simulink model "Mann_heat_transform"  (R2023a)
settings: Solver=VariableStepAuto  StartTime=0.0  StopTime=10.0  RelTol=1e-3
settings Model: Creator=bulldize  LastModifiedBy=bulldize

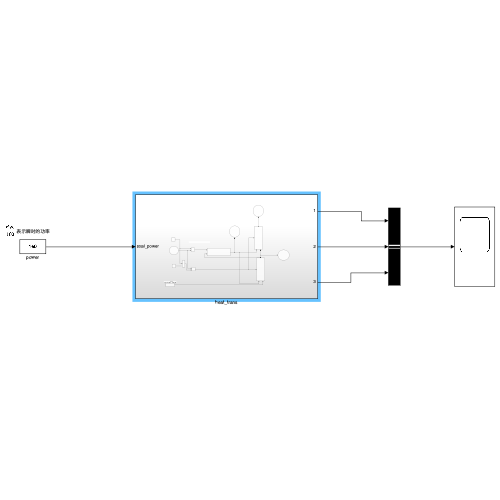
[thumbnail: Simulink's stored preview of the top-level diagram]
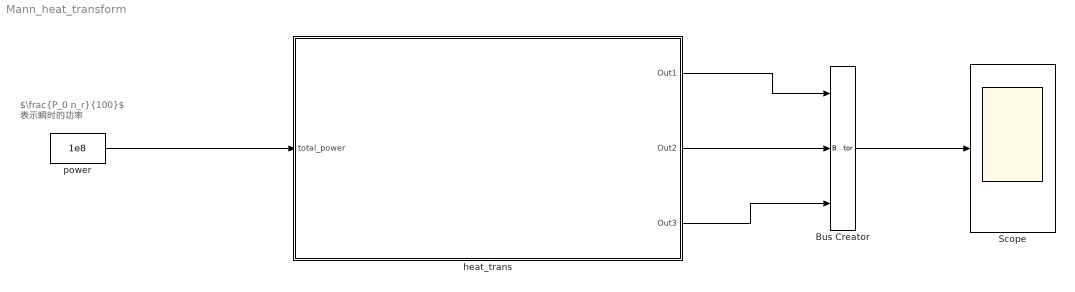
== system Mann_heat_transform ==
  note: $\frac{P_0 n_r}{100}$ 表示瞬时的功率
  Bus Creator : BusCreator  Inputs=3
  Scope : Scope
  heat_trans : Subsystem
  power : Constant  Value=1e8
  wires:
  power/1 -> heat_trans/1(total_power)
  heat_trans/1(Out1) -> Bus Creator/1
  heat_trans/2(Out2) -> Bus Creator/2
  heat_trans/3(Out3) -> Bus Creator/3
  Bus Creator/1 -> Scope/1

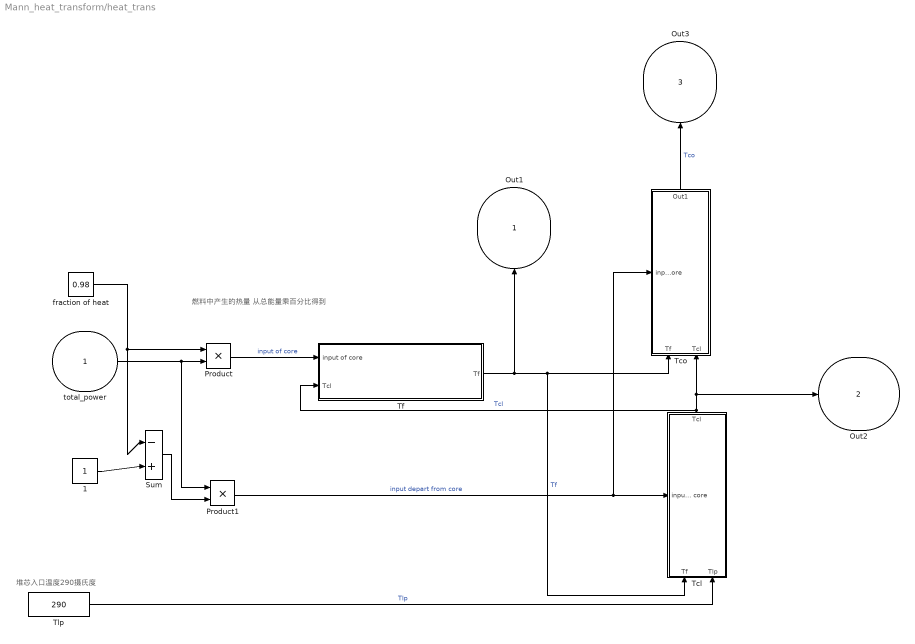
== system Mann_heat_transform/heat_trans ==
  note: 堆芯入口温度290摄氏度
  note: 燃料中产生的热量 从总能量乘百分比得到
  total_power : Inport
  1 : Constant
  Product : Product
  Product1 : Product
  Sum : Sum  Inputs=|-+
  Tcl : Subsystem
      settings: PortSchema="{\"entries\":[{\"content\":{\"sides\":[{\"content\":{\"connectorIds\":[\"In1\",\"In2\"]},\"type\":\"ConnectorPlacement.EquallySpacedRectSide\",\"uuid\":\"cb92287a-58d5-46bc-8bcc-fd7670e170d2\"},{\"content\":{\"connectorIds\":[\"Out1\"],\"side\":\"RIGHT\"},\"type\":\"ConnectorPlacement.EquallySpacedRectSide\",\"uuid\":\"3ab69de5-3a88-429e-9ba8-55afb0ea25a3\"},{\"content\":{\"connectorIds\":[\"In3\"],\"side\":\"TOP\"},\"type\":\"ConnectorPlacement.EquallySpacedRectSide\",\"uuid\":\"730caed0-fe0b-4665-bcfb-96be08a17aee\"}]},\"type\":\"ConnectorPlacement.EquallySpacedConnector\",\"uuid\":\"27471c3a-4cb2-4103-a1ca-5887cde1e89e\"}],\"packageUris\":[\"http://schema.mathworks.com/mf0/Connector/R2020b\"],\"version\":\"1.0\"}"
  Tco : Subsystem
      settings: PortSchema="{\"entries\":[{\"content\":{\"sides\":[{\"content\":{\"connectorIds\":[\"In1\",\"In2\"]},\"type\":\"ConnectorPlacement.EquallySpacedRectSide\",\"uuid\":\"cb92287a-58d5-46bc-8bcc-fd7670e170d2\"},{\"content\":{\"connectorIds\":[\"Out1\"],\"side\":\"RIGHT\"},\"type\":\"ConnectorPlacement.EquallySpacedRectSide\",\"uuid\":\"3ab69de5-3a88-429e-9ba8-55afb0ea25a3\"},{\"content\":{\"connectorIds\":[\"In3\"],\"side\":\"TOP\"},\"type\":\"ConnectorPlacement.EquallySpacedRectSide\",\"uuid\":\"730caed0-fe0b-4665-bcfb-96be08a17aee\"}]},\"type\":\"ConnectorPlacement.EquallySpacedConnector\",\"uuid\":\"27471c3a-4cb2-4103-a1ca-5887cde1e89e\"}],\"packageUris\":[\"http://schema.mathworks.com/mf0/Connector/R2020b\"],\"version\":\"1.0\"}"
  Tf : Subsystem
  Tlp : Constant  Value=290
  fraction of heat : Constant  Value=0.98
  Out1 : Outport
  Out2 : Outport  Port=2
  Out3 : Outport  Port=3
  wires:
  fraction of heat/1 -> Sum/1, Product/1
  total_power/1 -> Product1/1, Product/2
  1/1 -> Sum/2
  Sum/1 -> Product1/2
  Product/1 -> Tf/1(input of core)  "input of core"
  Tcl/1(Tcl) -> Tf/2(Tcl), Tco/2(Tcl), Out2/1  "Tcl"
  Tf/1(Tf) -> Tco/1(Tf), Tcl/1(Tf), Out1/1  "Tf"
  Tlp/1 -> Tcl/2(Tlp)  "Tlp"
  Product1/1 -> Tco/3(input depart from core), Tcl/3(input depart from core)  "input depart from core"
  Tco/1(Out1) -> Out3/1  "Tco"

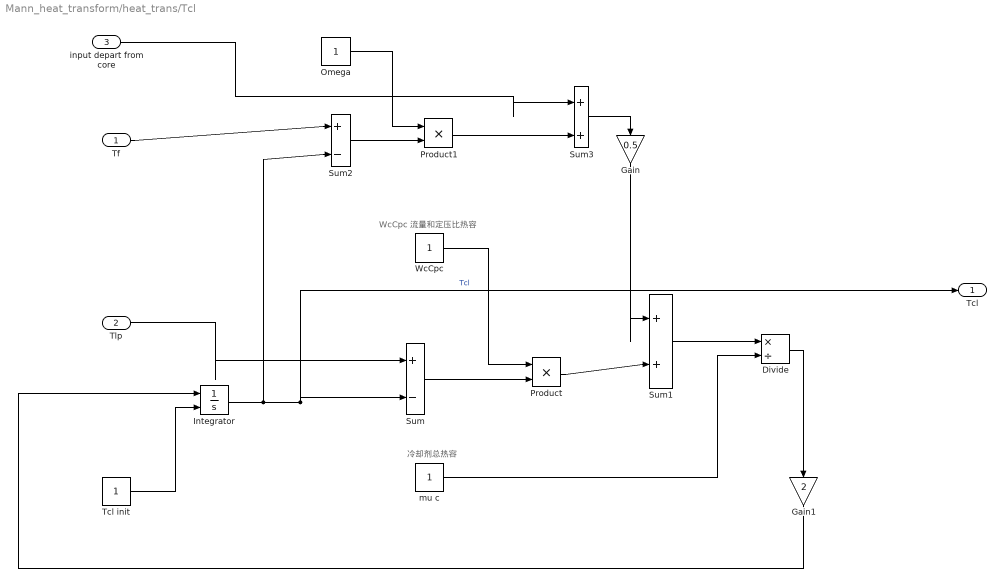
== system Mann_heat_transform/heat_trans/Tcl ==
  note: 冷却剂总热容
  note: WcCpc 流量和定压比热容
  Tf : Inport
  Tlp : Inport  Port=2
  input depart from core : Inport  Port=3
  Divide : Product  Inputs=*/
  Gain : Gain  Gain=0.5
  Gain1 : Gain  Gain=2
  Integrator : Integrator  InitialConditionSource=external
  Omega : Constant
  Product : Product
  Product1 : Product
  Sum : Sum  Inputs=|+-
  Sum1 : Sum  Inputs=|++
  Sum2 : Sum  Inputs=|+-
  Sum3 : Sum  Inputs=|++
  "Tcl init " : Constant
  WcCpc : Constant
  mu c : Constant
  Tcl : Outport
  wires:
  WcCpc/1 -> Product/1
  Product/1 -> Sum1/2
  "Tcl init "/1 -> Integrator/2
  Sum/1 -> Product/2
  Tlp/1 -> Sum/1
  Divide/1 -> Gain1/1
  Tf/1 -> Sum2/1
  Sum3/1 -> Gain/1
  mu c/1 -> Divide/2
  Integrator/1 -> Sum2/2, Tcl/1, Sum/2  "Tcl"
  Gain/1 -> Sum1/1
  Gain1/1 -> Integrator/1
  Sum1/1 -> Divide/1
  Omega/1 -> Product1/1
  Product1/1 -> Sum3/2
  Sum2/1 -> Product1/2
  input depart from core/1 -> Sum3/1

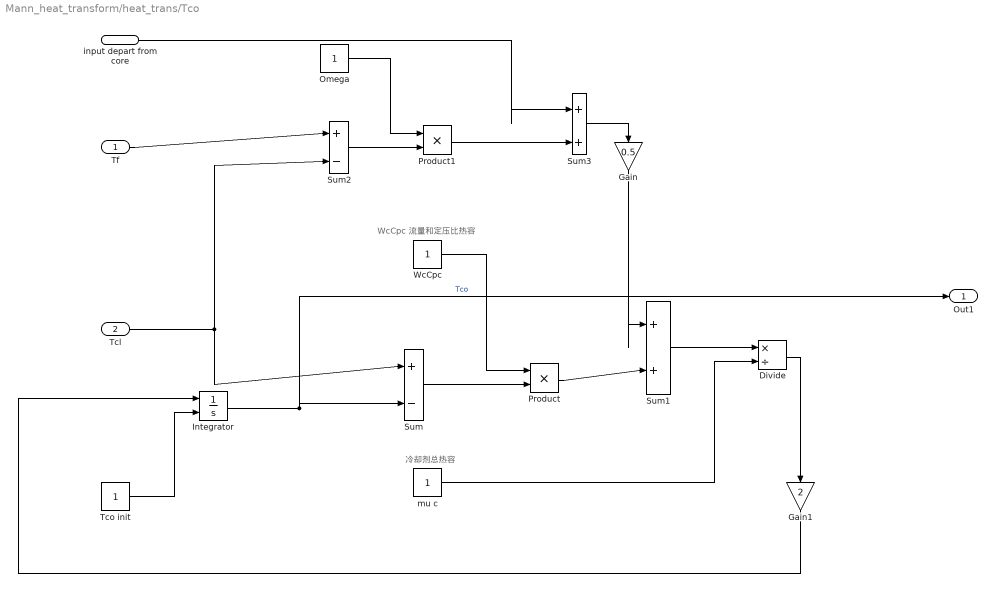
== system Mann_heat_transform/heat_trans/Tco ==
  note: 冷却剂总热容
  note: WcCpc 流量和定压比热容
  Tf : Inport
  Tcl : Inport  Port=2
  input depart from core : Inport  Port=3
  Divide : Product  Inputs=*/
  Gain : Gain  Gain=0.5
  Gain1 : Gain  Gain=2
  Integrator : Integrator  InitialConditionSource=external
  Omega : Constant
  Product : Product
  Product1 : Product
  Sum : Sum  Inputs=|+-
  Sum1 : Sum  Inputs=|++
  Sum2 : Sum  Inputs=|+-
  Sum3 : Sum  Inputs=|++
  "Tco init " : Constant
  WcCpc : Constant
  mu c : Constant
  Out1 : Outport
  wires:
  Integrator/1 -> Out1/1, Sum/2  "Tco"
  Sum1/1 -> Divide/1
  mu c/1 -> Divide/2
  Product/1 -> Sum1/2
  WcCpc/1 -> Product/1
  "Tco init "/1 -> Integrator/2
  Sum/1 -> Product/2
  Tcl/1 -> Sum/1, Sum2/2
  Tf/1 -> Sum2/1
  Omega/1 -> Product1/1
  Sum2/1 -> Product1/2
  input depart from core/1 -> Sum3/1
  Product1/1 -> Sum3/2
  Sum3/1 -> Gain/1
  Gain/1 -> Sum1/1
  Divide/1 -> Gain1/1
  Gain1/1 -> Integrator/1

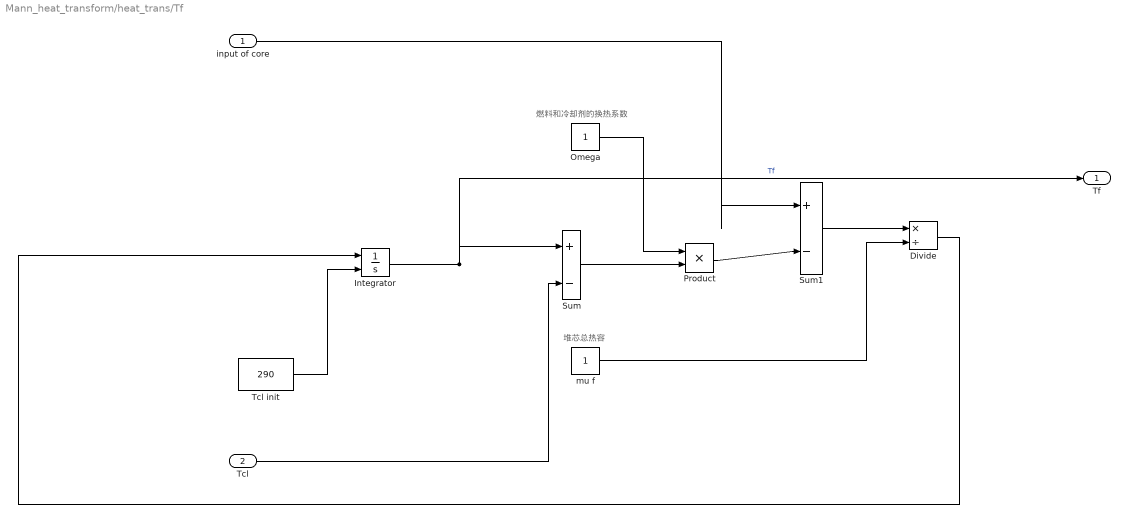
== system Mann_heat_transform/heat_trans/Tf ==
  note: 堆芯总热容
  note: 燃料和冷却剂的换热系数
  input of core : Inport
  Tcl : Inport  Port=2
  Divide : Product  Inputs=*/
  Integrator : Integrator  InitialConditionSource=external
  Omega : Constant
  Product : Product
  Sum : Sum  Inputs=|+-
  Sum1 : Sum  Inputs=|+-
  "Tcl init " : Constant  Value=290
  mu f : Constant
  Tf : Outport
  wires:
  Integrator/1 -> Tf/1, Sum/1  "Tf"
  Tcl/1 -> Sum/2
  Sum/1 -> Product/2
  Omega/1 -> Product/1
  Product/1 -> Sum1/2
  input of core/1 -> Sum1/1
  Sum1/1 -> Divide/1
  mu f/1 -> Divide/2
  Divide/1 -> Integrator/1
  "Tcl init "/1 -> Integrator/2
